simulink model "p4_simulinkk"  (R2025a)
settings: Solver=ode45  StartTime=0.0  StopTime=60  FixedStep=.01  MaxStep=0.01  RelTol=1e-3
values from neighbouring files (symbols this model uses):
  total_length = path.total_length    [gentrack.m]    (also in run_ev_sim.m)
  xpath = path.xpath    [gentrack.m]
  ypath = path.ypath    [gentrack.m]
undefined symbols (not defined in the file or in its folder): car, motor
settings Model: Creator=colto  LastModifiedBy=umar

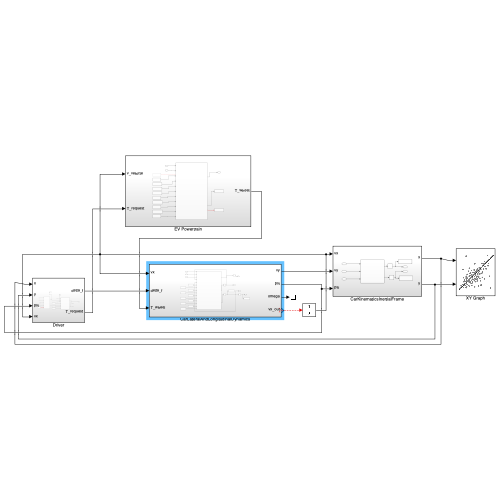
[thumbnail: Simulink's stored preview of the top-level diagram]
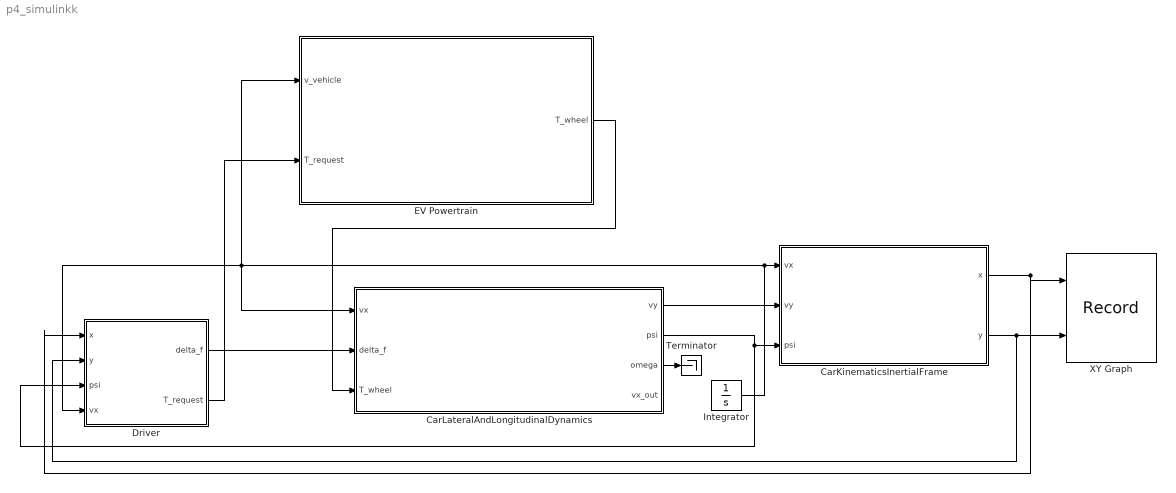
== system p4_simulinkk ==
  CarKinematicsInertialFrame : Subsystem
  CarLateralAndLongitudinalDynamics : Subsystem
  Driver : Subsystem
  EV Powertrain : Subsystem
  Integrator : Integrator
  Terminator : Terminator
  XY Graph : Record  NumPorts=2.0  FileSettingsInternal="{\"entries\":[{\"content\":{\"excelSettings\":{\"content\":{},\"type\":\"Streamout.ExcelSettings\"},\"parquetSettings\":{\"content\":{},\"type\":\"Streamout.ParquetSettings\"}},\"type\":\"Streamout.FileSettingStorage\",\"uuid\":\"\"}],\"packageUris\":[\"http:\\/\\/schema.mathworks.com\\/mf0\\/streamout_blocks\\/R2020a\"],\"version\":\"1.0\"}"  FrameSettings=[0, 0]  Layout=[1 1]  SignalsInternal="{\"entries\":[{\"content\":{\"signals\":[{\"content\":{\"blockPath\":[],\"dimensions\":[1],\"domain\":\"\",\"lineColor\":\"#a2142f\",\"plots\":[ 1 ],\"port\":1,\"sid\":[\"\"],\"signalID\":1,\"signalName\":\"CarKinematicsInertialFrame:1\"},\"type\":\"RecordBlkView.Signal\",\"uuid\":\"\"},{\"content\":{\"blockPath\":[],\"dimensions\":[1],\"domain\":\"\",\"lineColor\":\"#139fff\",\"plots\":[ 1 ],\"port\":2,\"sid\":[\"\"],\"signalID\":2,\"signalName\":\"CarKinematicsInertialFrame:2\"},\"type\":\"RecordBlkView.Signal\",\"uuid\":\"\"}]},\"type\":\"RecordBlkView.InputSignals\",\"uuid\":\"\"}],\"packageUris\":[\"http:\\/\\/schema.mathworks.com\\/mf0\\/streamout_blocks\\/R2020a\"],\"version\":\"1.0\"}"  VisualizationBindings="{\"xyplotplugin\":{\"info\":[{\"series\":[{\"bindingParametersList\":[{\"parameter\":\"X-Axis\",\"signalID\":1,\"signalName\":\"CarKinematicsInertialFrame:1\"},{\"parameter\":\"Y-Axis\",\"signalID\":2,\"signalName\":\"CarKinematicsInertialFrame:2\"}],\"seriesID\":0}],\"subplotID\":1}]}}"  CompatibilityTag=XY
  wires:
  CarKinematicsInertialFrame/1(x) -> XY Graph/1, Driver/1(x)
  CarKinematicsInertialFrame/2(y) -> Driver/2(y), XY Graph/2
  Driver/1(delta_f) -> CarLateralAndLongitudinalDynamics/2(delta_f)
  CarLateralAndLongitudinalDynamics/2(psi) -> Driver/3(psi), CarKinematicsInertialFrame/3(psi)
  CarLateralAndLongitudinalDynamics/1(vy) -> CarKinematicsInertialFrame/2(vy)
  ? -> Integrator/1
  Integrator/1 -> CarLateralAndLongitudinalDynamics/1(vx), Driver/4(vx), EV Powertrain/1(v_vehicle), CarKinematicsInertialFrame/1(vx)
  CarLateralAndLongitudinalDynamics/3(omega) -> Terminator/1
  EV Powertrain/1(T_wheel) -> CarLateralAndLongitudinalDynamics/3(T_wheel)
  Driver/2(T_request) -> EV Powertrain/2(T_request)

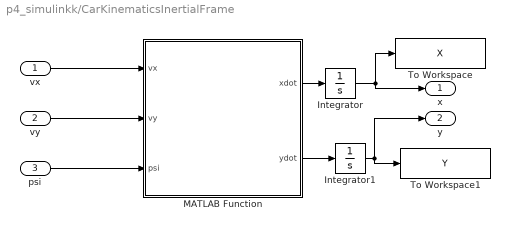
== system p4_simulinkk/CarKinematicsInertialFrame ==
  vx : Inport
  vy : Inport  Port=2
  psi : Inport  Port=3
  Integrator : Integrator  InitialCondition=car.init.X0
  Integrator1 : Integrator  InitialCondition=car.init.Y0
  MATLAB Function : MATLAB Function  TreatAsAtomicUnit=on
  To Workspace : ToWorkspace  VariableName=X  SaveFormat=Timeseries  SampleTime=-1
  To Workspace1 : ToWorkspace  VariableName=Y  SaveFormat=Timeseries  SampleTime=-1
  x : Outport
  y : Outport  Port=2
  wires:
  vx/1 -> MATLAB Function/1(vx)
  vy/1 -> MATLAB Function/2(vy)
  psi/1 -> MATLAB Function/3(psi)
  MATLAB Function/1(xdot) -> Integrator/1
  MATLAB Function/2(ydot) -> Integrator1/1
  Integrator/1 -> To Workspace/1, x/1
  Integrator1/1 -> y/1, To Workspace1/1

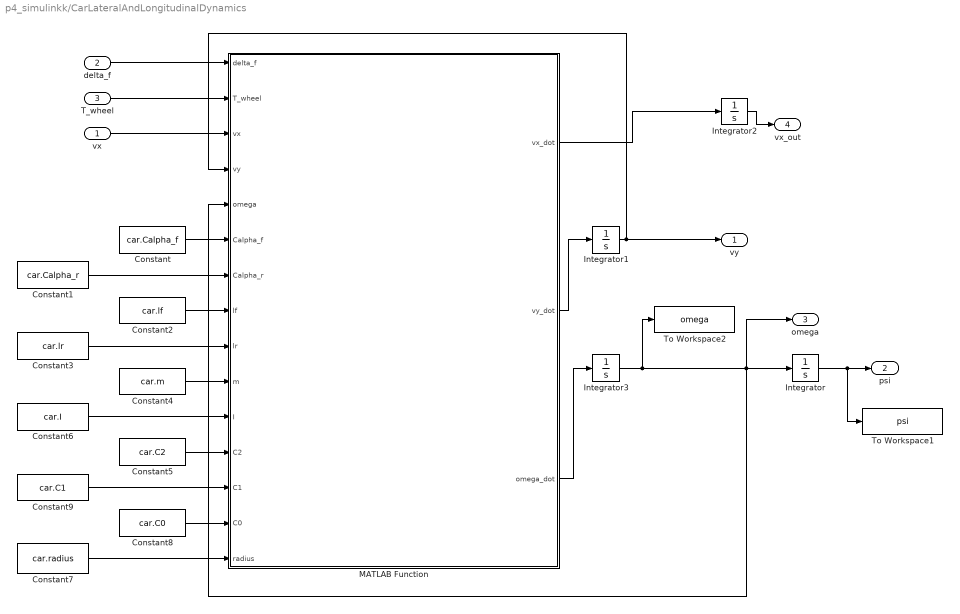
== system p4_simulinkk/CarLateralAndLongitudinalDynamics ==
  vx : Inport
  delta_f : Inport  Port=2
  T_wheel : Inport  Port=3
  Constant : Constant  Value=car.Calpha_f
  Constant1 : Constant  Value=car.Calpha_r
  Constant2 : Constant  Value=car.lf
  Constant3 : Constant  Value=car.lr
  Constant4 : Constant  Value=car.m
  Constant5 : Constant  Value=car.C2
  Constant6 : Constant  Value=car.I
  Constant7 : Constant  Value=car.radius
  Constant8 : Constant  Value=car.C0
  Constant9 : Constant  Value=car.C1
  Integrator{,1..3} (4 alike) : Integrator
  MATLAB Function : MATLAB Function  TreatAsAtomicUnit=on
  To Workspace1 : ToWorkspace  VariableName=psi  SaveFormat=Timeseries  SampleTime=-1
  To Workspace2 : ToWorkspace  VariableName=omega  SaveFormat=Timeseries  SampleTime=-1
  vy : Outport
  psi : Outport  Port=2
  omega : Outport  Port=3
  vx_out : Outport  Port=4
  wires:
  delta_f/1 -> MATLAB Function/1(delta_f)
  MATLAB Function/2(vy_dot) -> Integrator1/1
  Integrator1/1 -> MATLAB Function/4(vy), vy/1
  MATLAB Function/3(omega_dot) -> Integrator3/1
  Integrator3/1 -> To Workspace2/1, MATLAB Function/5(omega), Integrator/1, omega/1
  Integrator/1 -> To Workspace1/1, psi/1
  T_wheel/1 -> MATLAB Function/2(T_wheel)
  MATLAB Function/1(vx_dot) -> Integrator2/1
  vx/1 -> MATLAB Function/3(vx)
  Constant/1 -> MATLAB Function/6(Calpha_f)
  Constant1/1 -> MATLAB Function/7(Calpha_r)
  Constant2/1 -> MATLAB Function/8(lf)
  Constant3/1 -> MATLAB Function/9(lr)
  Constant4/1 -> MATLAB Function/10(m)
  Constant6/1 -> MATLAB Function/11(I)
  Constant5/1 -> MATLAB Function/12(C2)
  Constant9/1 -> MATLAB Function/13(C1)
  Constant8/1 -> MATLAB Function/14(C0)
  Constant7/1 -> MATLAB Function/15(radius)
  Integrator2/1 -> vx_out/1

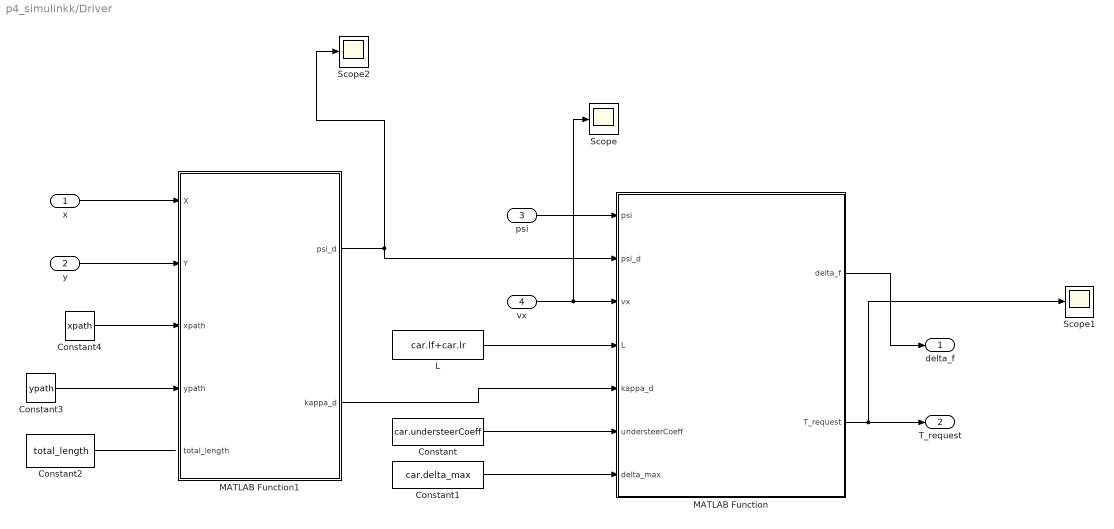
== system p4_simulinkk/Driver ==
  x : Inport
  y : Inport  Port=2
  psi : Inport  Port=3
  vx : Inport  Port=4
  Constant : Constant  Value=car.understeerCoeff
  Constant1 : Constant  Value=car.delta_max
  Constant2 : Constant  Value=total_length
  Constant3 : Constant  Value=ypath
  Constant4 : Constant  Value=xpath
  L : Constant  Value=car.lf+car.lr
  MATLAB Function : MATLAB Function  TreatAsAtomicUnit=on
  MATLAB Function1 : MATLAB Function  TreatAsAtomicUnit=on
  Scope : Scope
      settings: ActiveDisplayYMinimum=-10.267921415198117  ActiveDisplayYMaximum=55.451938980392029
  Scope1 : Scope
      settings: ActiveDisplayYMinimum=-1  ActiveDisplayYMaximum=1
  Scope2 : Scope
      settings: ActiveDisplayYMinimum=-0.067649021868334436  ActiveDisplayYMaximum=0.70836083516414972  DataLoggingVariableName=ScopeData2
  delta_f : Outport
  T_request : Outport  Port=2
  wires:
  x/1 -> MATLAB Function1/1(X)
  y/1 -> MATLAB Function1/2(Y)
  MATLAB Function/1(delta_f) -> delta_f/1
  psi/1 -> MATLAB Function/1(psi)
  MATLAB Function1/1(psi_d) -> Scope2/1, MATLAB Function/2(psi_d)
  L/1 -> MATLAB Function/4(L)
  vx/1 -> Scope/1, MATLAB Function/3(vx)
  MATLAB Function/2(T_request) -> Scope1/1, T_request/1
  Constant4/1 -> MATLAB Function1/3(xpath)
  Constant3/1 -> MATLAB Function1/4(ypath)
  Constant2/1 -> ?
  MATLAB Function1/2(kappa_d) -> MATLAB Function/5(kappa_d)
  Constant1/1 -> MATLAB Function/7(delta_max)
  Constant/1 -> MATLAB Function/6(understeerCoeff)

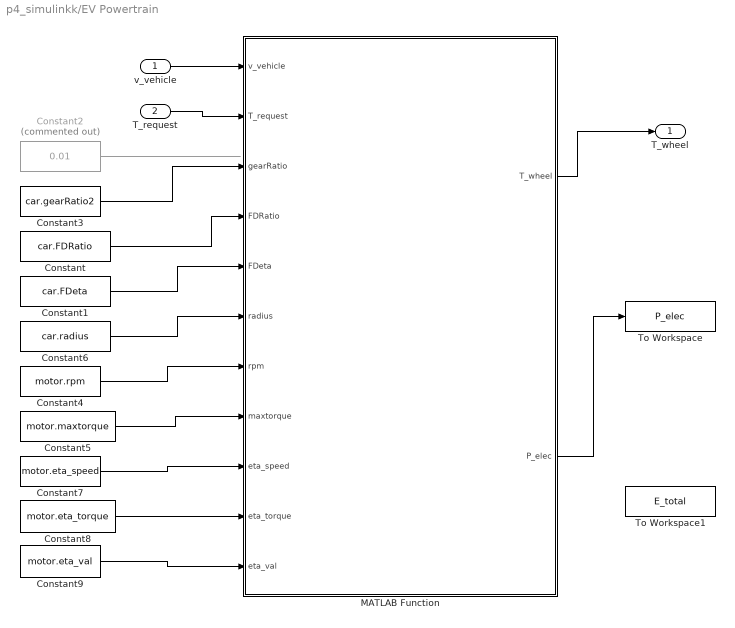
== system p4_simulinkk/EV Powertrain ==
  v_vehicle : Inport
  T_request : Inport  Port=2
  Constant : Constant  Value=car.FDRatio
  Constant1 : Constant  Value=car.FDeta
  Constant2 : Constant  Commented=on  Value=0.01
  Constant3 : Constant  Value=car.gearRatio2
  Constant4 : Constant  Value=motor.rpm
  Constant5 : Constant  Value=motor.maxtorque
  Constant6 : Constant  Value=car.radius
  Constant7 : Constant  Value=motor.eta_speed
  Constant8 : Constant  Value=motor.eta_torque
  Constant9 : Constant  Value=motor.eta_val
  MATLAB Function : MATLAB Function  TreatAsAtomicUnit=on
  To Workspace : ToWorkspace  VariableName=P_elec  SaveFormat=Timeseries  SampleTime=-1
  To Workspace1 : ToWorkspace  VariableName=E_total  SaveFormat=Timeseries  SampleTime=-1
  T_wheel : Outport
  wires:
  v_vehicle/1 -> MATLAB Function/1(v_vehicle)
  MATLAB Function/1(T_wheel) -> T_wheel/1
  T_request/1 -> MATLAB Function/2(T_request)
  MATLAB Function/2(P_elec) -> To Workspace/1
  ? -> To Workspace1/1
  Constant2/1 -> ?
  Constant3/1 -> MATLAB Function/3(gearRatio)
  Constant/1 -> MATLAB Function/4(FDRatio)
  Constant1/1 -> MATLAB Function/5(FDeta)
  Constant6/1 -> MATLAB Function/6(radius)
  Constant4/1 -> MATLAB Function/7(rpm)
  Constant5/1 -> MATLAB Function/8(maxtorque)
  Constant7/1 -> MATLAB Function/9(eta_speed)
  Constant9/1 -> MATLAB Function/11(eta_val)
  Constant8/1 -> MATLAB Function/10(eta_torque)

== matlab function p4_simulinkk/CarKinematicsInertialFrame/MATLAB Function ==
  data: vx input; xdot output; vy input; psi input; ydot output
function [xdot, ydot] = Kinematics(vx, vy, psi)
% Converts body-frame velocities (vx, vy) into inertial frame derivatives (xdot, ydot)
% Inputs:
%   vx  - longitudinal velocity in body frame (m/s)
%   vy  - lateral velocity in body frame (m/s)
%   psi - heading angle (rad)
% Outputs:
%   xdot - global X velocity (m/s)
%   ydot - global Y velocity (m/s)

% Rotation from body to inertial frame
R = [cos(psi), -sin(psi);
     sin(psi),  cos(psi)];

% Transform velocity vector
v_global = R * [vx; vy];

% Get components
xdot = v_global(1);
ydot = v_global(2);
end

== matlab function p4_simulinkk/Driver/MATLAB Function ==
  data: psi input; psi_d input; vx input; delta_f output; L input; T_request output; kappa_d input; understeerCoeff input; delta_max input
function [delta_f, T_request] = driver(psi, psi_d, vx, L, kappa_d, understeerCoeff, delta_max)
% Inputs:
%   psi             - current heading (rad)
%   psi_d           - desired heading from pure pursuit (rad)
%   vx              - actual longitudinal speed (m/s)
%   vxd             - desired longitudinal speed (m/s)
%   L               - wheelbase (m)
%   kappa_d         - desired curvature (1/m)
%   understeerCoeff - understeer gain (rad·s²/m²)
%   delta_max       - max steering angle (rad)
% Outputs:
%   delta_f         - steering angle (rad)
%   T_request       - requested drive torque (Nm)


vmax = 50; %change to desired max speed
Kkappa = 500;
vxd = max(5, vmax - Kkappa * abs(kappa_d));

% Controller gain
Kp_steer = 0.075;

% Heading error
e = psi_d - psi;

% Feedforward Ackermann steering
delta_ff = L * kappa_d;

% Understeer correction
delta_us = understeerCoeff * vx^2;

% Combined steering command
delta_f = Kp_steer * e + delta_ff + delta_us;

% Saturate steering angle
delta_f = min(max(delta_f, -delta_max), delta_max);

% --- Longitudinal Controller ---

% Proportional gain for torque control
Kp_torque = 2000;  % Nm per (m/s) of speed error 

% Speed error
speed_error = vxd - vx;

% Requested drive torque
T_request = Kp_torque * speed_error;

% Saturate torque to motor limits 
T_request = min(max(T_request, 0), 800);
end

== matlab function p4_simulinkk/EV Powertrain/MATLAB Function ==
  settings: updateMethod=DISCRETE
  data: v_vehicle input; T_wheel output; T_request input; gearRatio input; FDRatio input; P_elec output; FDeta input; radius input; rpm input; maxtorque input; eta_speed input; eta_torque input; eta_val input
%function [T_wheel, P_elec, E_total] = evPowertrain(v_vehicle, T_request, dt, gearRatio, FDRatio, FDeta, radius, rpm, maxtorque, eta_speed, eta_torque, eta_val)
% % EV Powertrain block for Simulink
% % Inputs:
% %   v_vehicle - vehicle speed (m/s)
% %   T_request - requested wheel torque (Nm)
% %   car       - struct from p4_init (car parameters)
% %   motor     - struct from p4_init (motor parameters)
% %   dt        - timestep (s)
% % Outputs:
% %   T_wheel   - delivered wheel torque (Nm)
% %   P_elec    - electrical power draw (W)
% %   E_total   - cumulative energy used (kWh)
% 
% persistent E_int
% if isempty(E_int)
%     E_int = 0;
% end
% 
% % Transmission parameters
% GR = gearRatio;
% FD = FDRatio;
% eta_fd = FDeta;
% 
% % Motor speed (rad/s → rpm)
% w_motor = (v_vehicle / radius) / (FD * GR);
% rpm_motor = w_motor * 60 / (2 * pi);
% 
% % Motor torque limit
% rpm_vec = rpm;
% %torque_max = interp1(rpm_vec, maxtorque(3,:), rpm_motor, 'linear', 'extrap');
% torque_max = interp1(rpm_vec, maxtorque, rpm_motor, 'linear', 'extrap');
% 
% % Requested motor torque
% T_motor_req = T_request / (GR * FD * eta_fd);
% 
% % Limit torque by motor capability
% T_motor = min(max(T_motor_req, -torque_max), torque_max);
% 
% % Motor efficiency
% eta = interp2(eta_speed, eta_torque, ...
%               eta_val, rpm_motor, abs(T_motor), 'linear', 0.9);
% 
% % Electrical power draw
% P_elec = abs(T_motor * w_motor / eta);
% if T_motor < 0
%     P_elec = 0; % No regen modeled yet
% end
% 
% % Energy tracking (in kWh)
% E_int = E_int + P_elec * dt;
% E_total = E_int / 3.6e6;
% 
% % Output wheel torque
% T_wheel = T_motor * GR * FD * eta_fd;
% end


function [T_wheel, P_elec] = evPowertrain(v_vehicle, T_request, gearRatio, FDRatio, FDeta, radius, rpm, maxtorque, eta_speed, eta_torque, eta_val)
% EV Powertrain block for Simulink
% Outputs:
%   T_wheel   - delivered wheel torque (Nm)
%   P_elec    - electrical power draw (W)

% Transmission parameters
GR = gearRatio;
FD = FDRatio;
eta_fd = FDeta;

% Motor speed (rad/s → rpm)
w_motor = (v_vehicle / radius) / (FD * GR);
rpm_motor = w_motor * 60 / (2 * pi);

% Motor torque limit
torque_max = interp1(rpm, maxtorque, rpm_motor, 'linear', 'extrap');

% Requested motor torque
T_motor_req = T_request / (GR * FD * eta_fd);

% Limit torque by motor capability
T_motor = min(max(T_motor_req, -torque_max), torque_max);

% Motor efficiency
eta = interp2(eta_speed, eta_torque, eta_val, rpm_motor, abs(T_motor), 'linear', 0.9);

% Electrical power draw
P_elec = abs(T_motor * w_motor / eta);
if T_motor < 0
    P_elec = 0; % No regen modeled yet
end

% Output wheel torque
T_wheel = T_motor * GR * FD * eta_fd;
end

== matlab function p4_simulinkk/CarLateralAndLongitudinalDynamics/MATLAB Function ==
  data: vx_dot output; delta_f input; T_wheel input; vx input; vy input; omega input; Calpha_f input; vy_dot output; omega_dot output; Calpha_r input; lf input; lr input; m input; I input; C2 input; C1 input; C0 input; radius input
function [vx_dot, vy_dot, omega_dot] = vehicleDynamics (delta_f, T_wheel, vx, vy, omega, Calpha_f, Calpha_r, lf, lr, m, I, C2, C1, C0, radius)

% Ensure minimum forward velocity to avoid division by zero
vx = max(vx, 0.1);

%% --- Lateral Dynamics ---
% Linear tire model
Fyf = -Calpha_f * (-delta_f - (vy + lf * omega) / vx);
Fyr = -Calpha_r * ((vy - lr * omega) / vx);

% Lateral acceleration
vy_dot = (Fyf + Fyr) / m - omega * vx;

% Yaw acceleration
omega_dot = (lf * Fyf - lr * Fyr) / I;

%% --- Longitudinal Dynamics ---
% Resistive forces
F_drag = C2 * vx^2;          % Aerodynamic drag
F_roll = C1 * vx + C0;       % Rolling resistance

% Driving force
F_drive = T_wheel / radius;

% Net force and acceleration
F_net = F_drive - F_drag - F_roll;
vx_dot = F_net / m;

end

== matlab function p4_simulinkk/Driver/MATLAB Function1 ==
  data: X input; psi_d output; Y input; xpath input; kappa_d output; ypath input; total_length input
function [psi_d, kappa_d] = PurePursuit(X, Y, xpath, ypath, total_length)
% Outputs desired heading and curvature

% Find closest point on path
distances = sqrt((xpath - X).^2 + (ypath - Y).^2);
[~, closestIdx] = min(distances);

% Lookahead logic
lookahead = 10; % Lookahead distance(m)
lookaheadIdx = min(closestIdx + round(lookahead / (total_length / length(xpath))), length(xpath));

% Target point
x_target = xpath(lookaheadIdx);
y_target = ypath(lookaheadIdx);

% Desired heading
dx = x_target - X;
dy = y_target - Y;
psi_d = atan2(dy, dx);

% Estimate curvature using finite difference
if lookaheadIdx > 1 && lookaheadIdx < length(xpath)
    dx1 = xpath(lookaheadIdx) - xpath(lookaheadIdx - 1);
    dy1 = ypath(lookaheadIdx) - ypath(lookaheadIdx - 1);
    dx2 = xpath(lookaheadIdx + 1) - xpath(lookaheadIdx);
    dy2 = ypath(lookaheadIdx + 1) - ypath(lookaheadIdx);

    angle1 = atan2(dy1, dx1);
    angle2 = atan2(dy2, dx2);
    dpsi = angle2 - angle1;
    ds = sqrt(dx1^2 + dy1^2);

    kappa_d = dpsi / ds;
else
    kappa_d = 0;
end
end
